simulink model "Lopez"  (R2021a)
settings: Solver=VariableStepAuto  StartTime=0.0  StopTime=100  RelTol=1e-3
settings Model: Creator=roberto  LastModifiedBy=Royer

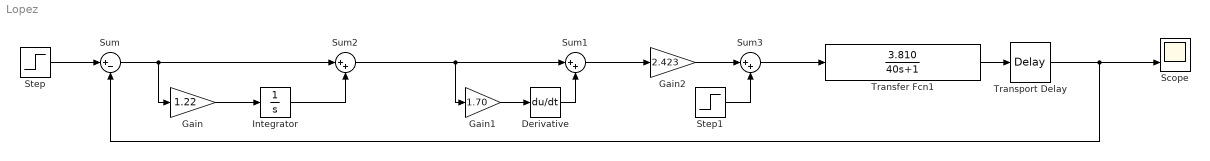
== system Lopez ==
  Derivative : Derivative
  Gain : Gain  Gain=1.22
  Gain1 : Gain  Gain=1.70
  Gain2 : Gain  Gain=2.423
  Integrator : Integrator
  Scope : Scope  NumInputPorts=2
  Step : Step  SampleTime=0
  Step1 : Step  SampleTime=0
  Sum : Sum  Inputs=|+-
  Sum1 : Sum  Inputs=|++
  Sum2 : Sum  Inputs=|++
  Sum3 : Sum  Inputs=|++
  Transfer Fcn1 : TransferFcn  Numerator=[3.810]  Denominator=[40 1]
  Transport Delay : TransportDelay  DelayTime=2.1
  wires:
  Step/1 -> Sum/1
  Gain1/1 -> Derivative/1
  Derivative/1 -> Sum1/2
  Sum1/1 -> Gain2/1
  Sum/1 -> Gain/1, Sum2/1
  Integrator/1 -> Sum2/2
  Gain/1 -> Integrator/1
  Sum2/1 -> Gain1/1, Sum1/1
  Gain2/1 -> Sum3/1
  Step1/1 -> Sum3/2
  Sum3/1 -> Transfer Fcn1/1
  Transfer Fcn1/1 -> Transport Delay/1
  Transport Delay/1 -> Sum/2, Scope/2
